simulink model "home_work_sim_01"  (R2023b)
settings: Solver=VariableStepAuto  StartTime=0.0  StopTime=10.0  MaxStep=0.001  RelTol=1e-3
libraries: simulink x1
settings Model: Creator=allso  LastModifiedBy=allso
settings SolverCC: AlgebraicLoopSolver=TrustRegion
settings DataIOCC: LimitDataPoints=on  SaveOutput=off  SaveTime=off
settings OptimizationCC: BlockReduction=off  BooleanDataType=off  LifeSpan=inf
settings DebuggingCC: SaveWithParameterizedLinksMsg=none  UnderspecifiedInitializationDetection=Classic  MergeDetectMultiDrivingBlocksExec=none  SignalResolutionControl=TryResolveAllWithWarning  UnconnectedInputMsg=warning  UnconnectedOutputMsg=warning  UnconnectedLineMsg=warning  AllowSymbolicDim=off  SFUnexpectedBacktrackingDiag=warning  SFNoUnconditionalDefaultTransitionDiag=warning  SFExecutionAtInitializationDiag=none  ArithmeticOperatorsInVariantConditions=warning
settings HardwareCC: TargetUnknown=on
settings ModelReferenceCC: EnableRefExpFcnMdlSchedulingChecks=on
settings SFSimCC: SimUseLocalCustomCode=off  CustomCodeUndefinedFunction=UseInterfaceOnly
settings RTWCC: RTWUseLocalCustomCode=off
settings CodeAppCC: StateflowObjectComments=on
settings GRTTargetCC: TargetLangStandard=C89/C90 (ANSI)

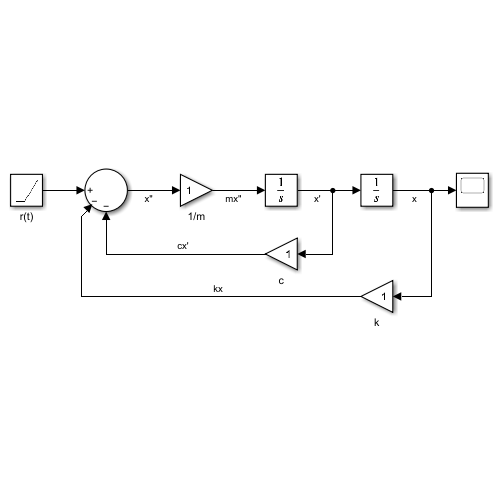
[thumbnail: Simulink's stored preview of the top-level diagram]
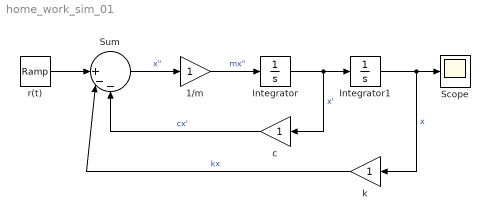
== system home_work_sim_01 ==
  1/m : Gain
  Integrator : Integrator
  Integrator1 : Integrator
  Scope : Scope
  Sum : Sum  Inputs=||+--
  c : Gain
  k : Gain
  r(t) : simulink/Sources/Ramp  slope=1  start=0  InitialOutput=0
  wires:
  Integrator/1 -> c/1, Integrator1/1  "x'"
  Sum/1 -> 1/m/1  "x\""
  Integrator1/1 -> k/1, Scope/1  "x"
  c/1 -> Sum/3  "cx'"
  k/1 -> Sum/2  "kx"
  1/m/1 -> Integrator/1  "mx\""
  r(t)/1 -> Sum/1
